simulink model "Lab3_M2V5_Motor_PositionControl_25a"  (R2025a)
settings: Solver=FixedStepDiscrete  StartTime=0.0  StopTime=inf  FixedStep=.004  RelTol=1e-3  EnableMultiTasking=on
libraries: arduinolib x2, arduinosensorlib x1
settings Model: SILPILModeSetting=veronly  ExtModeTrigDuration=2  Creator=hurstj  LastModifiedBy=hurstj
settings DataIOCC: SaveOutput=off  DSMLogging=off  SaveTime=off  ReturnWorkspaceOutputs=off
settings OptimizationCC: EnhancedBackFolding=on  PassReuseOutputArgsThreshold=0.0  MaxStackSize=64  OptimizeBlockOrder=speed  DifferentSizesBufferReuse=on  OptimizationCustomize=off
settings DebuggingCC: ParameterTunabilityLossMsg=error
settings HardwareCC: ProdBitPerInt=16.0  ProdBitPerPointer=16.0  ProdBitPerSizeT=16.0  ProdBitPerPtrDiffT=16.0  ProdLargestAtomicFloat=None  ProdWordSize=8.0  ProdHWDeviceType=Atmel->AVR  UseEmbeddedCoderFeatures=off  UseSimulinkCoderFeatures=off
settings ModelReferenceCC: EnableRefExpFcnMdlSchedulingChecks=on
settings SFSimCC: MATLABDynamicMemAlloc=off
settings RTWCC: SystemTargetFile=ert.tlc  HardwareBoard=Arduino Mega 2560  TemplateMakefile=ert_default_tmf  Toolchain=Arduino AVR  BuildConfiguration=Faster Runs  GPUComputeCapability=3.5  Description=Embedded Coder
settings CodeAppCC: ForceParamTrailComments=on  OperatorAnnotations=on
settings ERTTargetCC: ExtModeTransport=3.0  ExtModeStaticAllocSize=2048.0  InlinedParameterPlacement=Hierarchical  DynamicArrayContainerType=coder::array  ERTCustomFileBanners=off  SupportContinuousTime=on  SupportNonInlinedSFcns=on  RemoveResetFunc=off  SupportVariableSizeSignals=on  ModelStepFunctionPrototypeControlCompliant=off

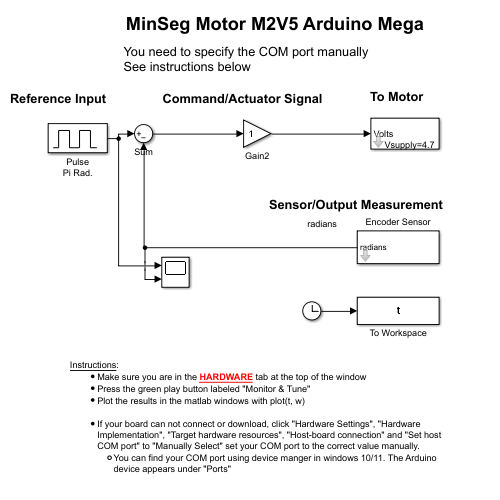
[thumbnail: Simulink's stored preview of the top-level diagram]
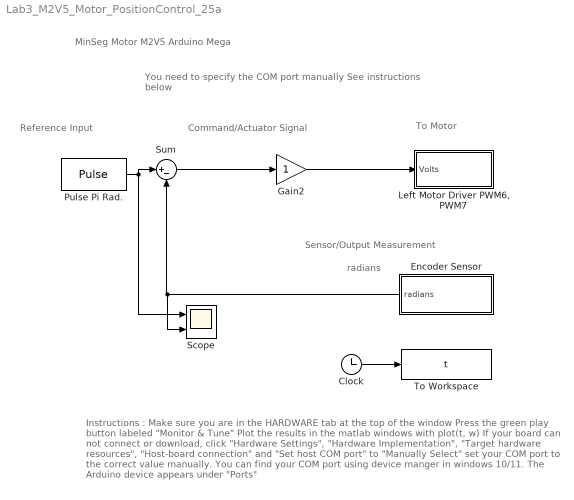
== system Lab3_M2V5_Motor_PositionControl_25a ==
  note: You need to specify the COM port manually
      | See instructions below
  note: Instructions :
      | Make sure you are in the HARDWARE tab at the top of the window
      | Press the green play button labeled "Monitor & Tune"
      | Plot the results in the matlab windows with plot(t, w)
      |
      | If your board can not connect or download, click "Hardware Settings", "Hardware Implementation", "Target hardware resources", "Host-board connection" and "Set host COM port" to "Manually Select" set your COM port to the correct value manually.
      | You can find your COM port using device manger in windows 10/11. The Arduino device appears under "Ports"
  note: MinSeg Motor M2V5 Arduino Mega
  note: Command/Actuator Signal
  note: radians
  note: Reference Input
  note: Sensor/Output Measurement
  note: To Motor
  Clock : Clock
  Encoder Sensor : Subsystem
      mask DialogControl Control2 Prompt: Encoder Counter - unknown units
  Gain2 : Gain
  "Left Motor Driver PWM6, PWM7" : Subsystem  mask{Vsupply=4.7, Voffset=0}
      mask prompts: Vsupply "Driver Voltage"; Voffset "Voltage offset (0-Vsupply)"
      mask help:
      | Specify driver supply voltage (3.9 for USB)
      | Specify the PWM offset (0-255)
      mask Display:
      | port_label('input',1,'Volts')
      | text(15,5,['Vsupply=' num2str(Vsupply)])
  Pulse Pi Rad. : DiscretePulseGenerator  PulseType=Time based  Amplitude=pi  Period=4  PulseWidth=50
  Scope : Scope  NumInputPorts=2
      settings: ActiveDisplayYMinimum=-1.3197746202349663  ActiveDisplayYMaximum=4.4002285525202751
  Sum : Sum  Inputs=|+-
  To Workspace : ToWorkspace  VariableName=t  SampleTime=-1
      settings: Save2DSignal=2-D array (concatenate along first dimension)
  wires:
  Encoder Sensor/1(radians) -> Scope/2, Sum/2
  Gain2/1 -> "Left Motor Driver PWM6, PWM7"/1(Volts)
  Clock/1 -> To Workspace/1
  Sum/1 -> Gain2/1
  Pulse Pi Rad./1 -> Sum/1, Scope/1

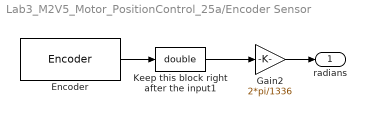
== system Lab3_M2V5_Motor_PositionControl_25a/Encoder Sensor ==
  Encoder : arduinosensorlib/Encoder  InputA=2  InputB=3  Mode=No reset  SampleTime=-1
  Gain2 : Gain  Gain=2*pi/1336
  Keep this block right after the input1 : DataTypeConversion  OutDataTypeStr=double  SaturateOnIntegerOverflow=off  RndMeth=Floor
  radians : Outport
  wires:
  Keep this block right after the input1/1 -> Gain2/1
  Gain2/1 -> radians/1
  Encoder/1 -> Keep this block right after the input1/1

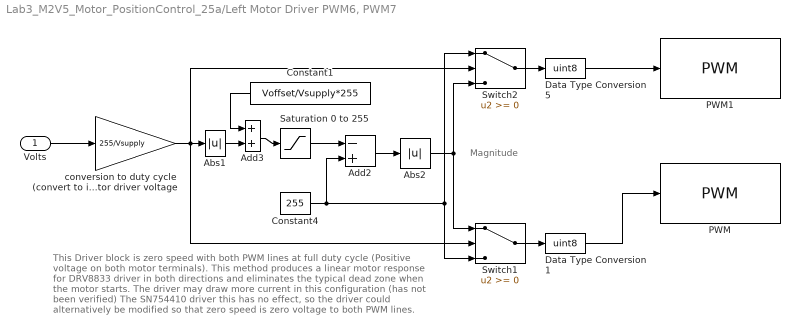
== system Lab3_M2V5_Motor_PositionControl_25a/Left Motor Driver PWM6, PWM7 ==
  note: Magnitude
  note: This Driver block is zero speed with both PWM lines at full duty cycle
      |  (Positive voltage on both motor terminals).
      | This method produces a linear motor response for DRV8833 driver
      |  in both directions and eliminates
      | the typical dead zone when the motor starts.
      | The driver may draw more current in this configuration (has not been verified)
      |
      | The SN754410 driver this has no effect, so the driver could alternatively
      | be modified so that zero speed is zero voltage to both PWM lines.
  Volts : Inport
  Abs1 : Abs  SaturateOnIntegerOverflow=off
  Abs2 : Abs  SaturateOnIntegerOverflow=off
  Add2 : Sum  Inputs=-+
  Add3 : Sum
  Constant1 : Constant  Value=Voffset/Vsupply*255
  Constant4 : Constant  Value=255
  Data Type Conversion1 : DataTypeConversion  OutDataTypeStr=uint8  SaturateOnIntegerOverflow=off  RndMeth=Floor
  Data Type Conversion5 : DataTypeConversion  OutDataTypeStr=uint8  SaturateOnIntegerOverflow=off  RndMeth=Floor
  PWM : arduinolib/PWM  pinNumber=7  frequencyType=Specify  desiredFrequency=32000  achievableFrequency=32000
  PWM1 : arduinolib/PWM  pinNumber=6  frequencyType=Specify  desiredFrequency=32000  achievableFrequency=32000
  Saturation 0 to 255 : Saturate  UpperLimit=255  LowerLimit=0
  Switch1 : Switch  SaturateOnIntegerOverflow=off  InputSameDT=off
  Switch2 : Switch  SaturateOnIntegerOverflow=off  InputSameDT=off
  conversion to duty cycle (convert to int) denominator is motor driver voltage : Gain  Gain=255/Vsupply  OutDataTypeStr=int16
  wires:
  Data Type Conversion1/1 -> PWM/1
  Data Type Conversion5/1 -> PWM1/1
  Switch1/1 -> Data Type Conversion1/1
  Switch2/1 -> Data Type Conversion5/1
  Abs2/1 -> Switch1/1, Switch2/3
  Add2/1 -> Abs2/1
  Constant4/1 -> Add2/2, Switch2/1, Switch1/3
  Saturation 0 to 255/1 -> Add2/1
  conversion to duty cycle (convert to int) denominator is motor driver voltage/1 -> Abs1/1, Switch2/2, Switch1/2
  Abs1/1 -> Add3/2
  Constant1/1 -> Add3/1
  Add3/1 -> Saturation 0 to 255/1
  Volts/1 -> conversion to duty cycle (convert to int) denominator is motor driver voltage/1
